simulink model "k1visitmyp"  (Simulink 8.8)
settings: Solver=ode45  StartTime=0.0  StopTime=10.0  RelTol=1e-3  EnableMultiTasking=on
libraries: cdsIPCx x26, cdsCDI64 x6, cdsCDO64 x6, BIO_CD_DECODE_MASTER x6, BIO_CD_ENCODE_MASTER x5, CHK_DIO x5, dac x3, cdsBit2Word x2, cdsAdcx0 x1, cdsAdcx1 x1, TYPEA_MASTER x1, cdsEpicsOut x1
settings Model: SuppressorTable=22 serialization::archive 11 0 3 0 0 0 11 0  Creator=controls  LastModifiedBy=controls
settings DataIOCC: SignalLoggingSaveFormat=Dataset
settings DebuggingCC: UnderspecifiedInitializationDetection=Simplified  MergeDetectMultiDrivingBlocksExec=error  FcnCallInpInsideContextMsg=error  AllowSymbolicDim=off  StateNameClashWarn=none
settings GRTTargetCC: CombineOutputUpdateFcns=on  GRTInterface=off

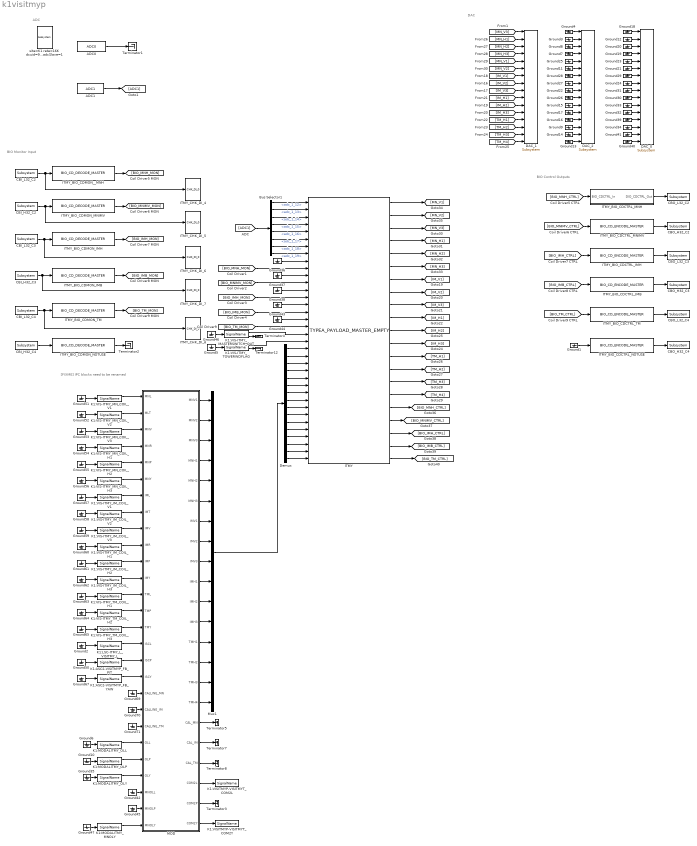
== system k1visitmyp ==
  note: [FIXME] IPC blocks need to be renamed
  note: BIO Monitor Input
  note: BIO Control Outputs
  note: DAC
  note: ADC
  ADC0 : cdsAdcx0/ADC0  Tag=cdsAdc  Description=|
      | type-GSC_16AI64SSA
      | card_num=0
      settings: AttributesFormatString=%<Description>\n%<Tag>
  ADC1 : cdsAdcx1/ADC1  Tag=cdsAdc  Description=|
      | type-GSC_16AI64SSA
      | card_num=1
      settings: AttributesFormatString=%<Description>\n%<Tag>
  Bus Selector1 : BusSelector  OutputSignals=adc_1_12,adc_1_13,adc_1_14,adc_1_15,adc_1_16,adc_1_17,adc_1_18,adc_1_19
  CBI_H32_C2 : cdsCDI64/Subsystem  Tag=cdsCDI64  Description=card_num=5
      settings: AttributesFormatString=%<Tag>\n%<Description>
  CBI_H32_C3 : cdsCDI64/Subsystem  Tag=cdsCDI64  Description=card_num=7
      settings: AttributesFormatString=%<Tag>\n%<Description>
  CBI_H32_C4 : cdsCDI64/Subsystem  Tag=cdsCDI64  Description=card_num=9
      settings: AttributesFormatString=%<Tag>\n%<Description>
  CBI_L32_C2 : cdsCDI64/Subsystem  Tag=cdsCDI64  Description=card_num=4
      settings: AttributesFormatString=%<Tag>\n%<Description>
  CBI_L32_C3 : cdsCDI64/Subsystem  Tag=cdsCDI64  Description=card_num=6
      settings: AttributesFormatString=%<Tag>\n%<Description>
  CBI_L32_C4 : cdsCDI64/Subsystem  Tag=cdsCDI64  Description=card_num=8
      settings: AttributesFormatString=%<Tag>\n%<Description>
  CBO_H32_C2 : cdsCDO64/Subsystem  Tag=cdsCDO64  Description=card_num=5
      settings: AttributesFormatString=%<Tag>\n%<Description>
  CBO_H32_C3 : cdsCDO64/Subsystem  Tag=cdsCDO64  Description=card_num=7
      settings: AttributesFormatString=%<Tag>\n%<Description>
  CBO_H32_C4 : cdsCDO64/Subsystem  Tag=cdsCDO64  Description=card_num=9
      settings: AttributesFormatString=%<Tag>\n%<Description>
  CBO_L32_C2 : cdsCDO64/Subsystem  Tag=cdsCDO64  Description=card_num=4
      settings: AttributesFormatString=%<Tag>\n%<Description>
  CBO_L32_C3 : cdsCDO64/Subsystem  Tag=cdsCDO64  Description=card_num=6
      settings: AttributesFormatString=%<Tag>\n%<Description>
  CBO_L32_C4 : cdsCDO64/Subsystem  Tag=cdsCDO64  Description=card_num=8
      settings: AttributesFormatString=%<Tag>\n%<Description>
  DAC_0 : dac/Subsystem  Description=|
      | type=GSC_16AO16,
      | card_num=0
      settings: AttributesFormatString=%<Description>
  DAC_1 : dac/Subsystem  Description=|
      | type=GSC_16AO16,
      | card_num=1
      settings: AttributesFormatString=%<Description>
  DAC_2 : dac/Subsystem  Description=|
      | type=GSC_16AO16,
      | card_num=2
      settings: AttributesFormatString=%<Description>
  Demux : Demux  Outputs=16
  Ground{1..47,50..65,67,69..71} (67 alike) : Ground
  ITMY : TYPEA_MASTER/TYPEA_PAYLOAD_MASTER_EMPTY
  ITMY_BIO_CDCTRL_IMB : BIO_CD_ENCODE_MASTER/BIO_CD_ENCODE_MASTER
  ITMY_BIO_CDCTRL_IMH : BIO_CD_ENCODE_MASTER/BIO_CD_ENCODE_MASTER
  ITMY_BIO_CDCTRL_MNH : Subsystem
  ITMY_BIO_CDCTRL_MNIMV : BIO_CD_ENCODE_MASTER/BIO_CD_ENCODE_MASTER
  ITMY_BIO_CDCTRL_NOTUSE : BIO_CD_ENCODE_MASTER/BIO_CD_ENCODE_MASTER
  ITMY_BIO_CDCTRL_TM : BIO_CD_ENCODE_MASTER/BIO_CD_ENCODE_MASTER
  ITMY_BIO_CDMON_IMB : BIO_CD_DECODE_MASTER/BIO_CD_DECODE_MASTER
  ITMY_BIO_CDMON_IMH : BIO_CD_DECODE_MASTER/BIO_CD_DECODE_MASTER
  ITMY_BIO_CDMON_MNIMV : BIO_CD_DECODE_MASTER/BIO_CD_DECODE_MASTER
  ITMY_BIO_CDMON_NOTUSE : BIO_CD_DECODE_MASTER/BIO_CD_DECODE_MASTER
  ITMY_BIO_CDMON_TM : BIO_CD_DECODE_MASTER/BIO_CD_DECODE_MASTER
  ITMY_BIO_CDMON__MNH : BIO_CD_DECODE_MASTER/BIO_CD_DECODE_MASTER
  ITMY_CHK_DI_{4..8} (5 alike) : CHK_DIO/CHK_DI_0
  K1:ASC2-VISITMYP_FB_PIT : cdsIPCx/SignalName  Tag=cdsIPCx_RFM  Description=card=1
      settings: AttributesFormatString=%<Description>\n%<Tag>
  K1:ASC2-VISITMYP_FB_YAW : cdsIPCx/SignalName  Tag=cdsIPCx_RFM  Description=card=1
      settings: AttributesFormatString=%<Description>\n%<Tag>
  K1:LSC-ITMY_L_VISITMY_L : cdsIPCx/SignalName  Tag=cdsIPCx_RFM  Description=card=1
      settings: AttributesFormatString=%<Description>\n%<Tag>
  K1:MODALITMY_MNOLY : cdsIPCx/SignalName  Tag=cdsIPCx_SHMEM  Description=Inter-Process Communication via Shared memory.
      settings: AttributesFormatString=%<Tag>
  K1:MODALITMY_OLL : cdsIPCx/SignalName  Tag=cdsIPCx_SHMEM  Description=Inter-Process Communication via Shared memory.
      settings: AttributesFormatString=%<Tag>
  K1:MODALITMY_OLP : cdsIPCx/SignalName  Tag=cdsIPCx_SHMEM  Description=Inter-Process Communication via Shared memory.
      settings: AttributesFormatString=%<Tag>
  K1:MODALITMY_OLY : cdsIPCx/SignalName  Tag=cdsIPCx_SHMEM  Description=Inter-Process Communication via Shared memory.
      settings: AttributesFormatString=%<Tag>
  K1:VIS-ITMY_IM_COIL_H1 : cdsIPCx/SignalName  Tag=cdsIPCx_SHMEM  Description=Inter-Process Communication via Shared memory.
      settings: AttributesFormatString=%<Tag>
  K1:VIS-ITMY_IM_COIL_H2 : cdsIPCx/SignalName  Tag=cdsIPCx_SHMEM  Description=Inter-Process Communication via Shared memory.
      settings: AttributesFormatString=%<Tag>
  K1:VIS-ITMY_IM_COIL_H3 : cdsIPCx/SignalName  Tag=cdsIPCx_SHMEM  Description=Inter-Process Communication via Shared memory.
      settings: AttributesFormatString=%<Tag>
  K1:VIS-ITMY_IM_COIL_V1 : cdsIPCx/SignalName  Tag=cdsIPCx_SHMEM  Description=Inter-Process Communication via Shared memory.
      settings: AttributesFormatString=%<Tag>
  K1:VIS-ITMY_IM_COIL_V2 : cdsIPCx/SignalName  Tag=cdsIPCx_SHMEM  Description=Inter-Process Communication via Shared memory.
      settings: AttributesFormatString=%<Tag>
  K1:VIS-ITMY_IM_COIL_V3 : cdsIPCx/SignalName  Tag=cdsIPCx_SHMEM  Description=Inter-Process Communication via Shared memory.
      settings: AttributesFormatString=%<Tag>
  K1:VIS-ITMY_MASTERSWITCH_OUT : cdsIPCx/SignalName  Tag=cdsIPCx_SHMEM  Description=Inter-Process Communication via Shared memory.
      settings: AttributesFormatString=%<Tag>
  K1:VIS-ITMY_MN_COIL_H1 : cdsIPCx/SignalName  Tag=cdsIPCx_SHMEM  Description=Inter-Process Communication via Shared memory.
      settings: AttributesFormatString=%<Tag>
  K1:VIS-ITMY_MN_COIL_H2 : cdsIPCx/SignalName  Tag=cdsIPCx_SHMEM  Description=Inter-Process Communication via Shared memory.
      settings: AttributesFormatString=%<Tag>
  K1:VIS-ITMY_MN_COIL_H3 : cdsIPCx/SignalName  Tag=cdsIPCx_SHMEM  Description=Inter-Process Communication via Shared memory.
      settings: AttributesFormatString=%<Tag>
  K1:VIS-ITMY_MN_COIL_V1 : cdsIPCx/SignalName  Tag=cdsIPCx_SHMEM  Description=Inter-Process Communication via Shared memory.
      settings: AttributesFormatString=%<Tag>
  K1:VIS-ITMY_MN_COIL_V2 : cdsIPCx/SignalName  Tag=cdsIPCx_SHMEM  Description=Inter-Process Communication via Shared memory.
      settings: AttributesFormatString=%<Tag>
  K1:VIS-ITMY_MN_COIL_V3 : cdsIPCx/SignalName  Tag=cdsIPCx_SHMEM  Description=Inter-Process Communication via Shared memory.
      settings: AttributesFormatString=%<Tag>
  K1:VIS-ITMY_TM_COIL_H1 : cdsIPCx/SignalName  Tag=cdsIPCx_SHMEM  Description=Inter-Process Communication via Shared memory.
      settings: AttributesFormatString=%<Tag>
  K1:VIS-ITMY_TM_COIL_H2 : cdsIPCx/SignalName  Tag=cdsIPCx_SHMEM  Description=Inter-Process Communication via Shared memory.
      settings: AttributesFormatString=%<Tag>
  K1:VIS-ITMY_TM_COIL_H3 : cdsIPCx/SignalName  Tag=cdsIPCx_SHMEM  Description=Inter-Process Communication via Shared memory.
      settings: AttributesFormatString=%<Tag>
  K1:VIS-ITMY_TOWERWDFLAG : cdsIPCx/SignalName  Tag=cdsIPCx_SHMEM  Description=Inter-Process Communication via Shared memory.
      settings: AttributesFormatString=%<Tag>
  K1:VISITMYP-VISITMYT_COM2L : cdsIPCx/SignalName  Tag=cdsIPCx_SHMEM  Description=Inter-Process Communication via Shared memory.
      settings: AttributesFormatString=%<Tag>
  K1:VISITMYP-VISITMYT_COM2Y : cdsIPCx/SignalName  Tag=cdsIPCx_SHMEM  Description=Inter-Process Communication via Shared memory.
      settings: AttributesFormatString=%<Tag>
  MOD : Subsystem  Tag=top_names
  Mux1 : Mux  Inputs=16
  Terminator{1..5,7..8,12} (8 alike) : Terminator
  site=K1 rate=16K dcuid=98 host=k1iy1 specific_cpu=3 adcSlave=1 : cdsParameters/Subsystem  Tag=cdsParameters  Description=|
      | Purpose:                                                                                                                                                                                                                                
      | Provide system parameters to the FE code generator to properly configure the generated EPICS names, rep rate of the FE controller, and the Data Acquisition node ID for proper storage of data from this FE controller.                 
      |                                                                                                                                                                                                                                         
      | Useage:                                                                                                                                                                                                                                 
      | The part NAME field is used to identify the FE parameters. It must be of the form:                                                                                                                                                      
      | site=                                                                                                                                                                                                                                   
      | rate=                                                                                                                                                                                                                                   
      | dcuid=                                                                                                                                                                                                                                  
      |                                                                                                                                                                                                                                         
      | Where:                                                                                                                                                                                                                                  
      | site= argument may be H1, H2, L1, M1, G1, either as a single argument or multiple, for example site=H1,H2. These are the only names allowed. These will become the first two characters of all EPICS and signal names (for example G1:).
      |                                                                                                                                                                                                                                         
      | rate= may be 2K, 16K, 32K, or 64K                                                                                                                                                                                                       
      |                                                                                                                                                                                                                                         
      | dcuid= is site specific ie it must be unique at each site.
      settings: AttributesFormatString=%<Tag>
  wires:
  ADC1/1 -> [ADC1]
  [MN_V3] -> DAC_1/1
  [MN_H1] -> DAC_1/2
  [MN_H2] -> DAC_1/3
  [MN_H3] -> DAC_1/4
  [MN_V1] -> DAC_1/5
  [MN_V2] -> DAC_1/6
  [IM_V1] -> DAC_1/7
  [IM_V2] -> DAC_1/8
  [IM_V3] -> DAC_1/9
  [IM_H1] -> DAC_1/10
  [TM_H1] -> DAC_1/13
  [TM_H4] -> DAC_1/16
  [TM_H3] -> DAC_1/15
  [TM_H2] -> DAC_1/14
  [IM_H2] -> DAC_1/11
  [IM_H3] -> DAC_1/12
  [BIO_MNH_CTRL] -> ITMY_BIO_CDCTRL_MNH/1(BIO_CDCTRL_In)
  ITMY_BIO_CDCTRL_MNH/1(DIO_CDCTRL_Out) -> CBO_L32_C2/1
  [BIO_MNIMV_CTRL] -> ITMY_BIO_CDCTRL_MNIMV/1
  ITMY_BIO_CDCTRL_MNIMV/1 -> CBO_H32_C2/1
  [BIO_IMH_CTRL] -> ITMY_BIO_CDCTRL_IMH/1
  ITMY_BIO_CDCTRL_IMH/1 -> CBO_L32_C3/1
  [BIO_IMB_CTRL] -> ITMY_BIO_CDCTRL_IMB/1
  ITMY_BIO_CDCTRL_IMB/1 -> CBO_H32_C3/1
  [BIO_TM_CTRL] -> ITMY_BIO_CDCTRL_TM/1
  ITMY_BIO_CDCTRL_TM/1 -> CBO_L32_C4/1
  Ground1/1 -> ITMY_BIO_CDCTRL_NOTUSE/1
  ITMY_BIO_CDCTRL_NOTUSE/1 -> CBO_H32_C4/1
  CBI_L32_C2/1 -> ITMY_CHK_DI_4/1, ITMY_BIO_CDMON__MNH/1
  ITMY_BIO_CDMON__MNH/1 -> [BIO_MNH_MON]
  CBI_H32_C2/1 -> ITMY_CHK_DI_5/1, ITMY_BIO_CDMON_MNIMV/1
  ITMY_BIO_CDMON_MNIMV/1 -> [BIO_MNIMV_MON]
  CBI_L32_C3/1 -> ITMY_CHK_DI_6/1, ITMY_BIO_CDMON_IMH/1
  ITMY_BIO_CDMON_IMH/1 -> [BIO_IMH_MON]
  ITMY_BIO_CDMON_IMB/1 -> [BIO_IMB_MON]
  CBI_L32_C4/1 -> ITMY_CHK_DI_8/1, ITMY_BIO_CDMON_TM/1
  ITMY_BIO_CDMON_TM/1 -> [BIO_TM_MON]
  CBI_H32_C4/1 -> ITMY_BIO_CDMON_NOTUSE/1
  ITMY_BIO_CDMON_NOTUSE/1 -> Terminator2/1
  Ground4/1 -> DAC_2/1
  Ground3/1 -> DAC_2/2
  Ground8/1 -> DAC_2/3
  Ground7/1 -> DAC_2/4
  Ground25/1 -> DAC_2/5
  Ground11/1 -> DAC_2/6
  Ground28/1 -> DAC_2/7
  Ground27/1 -> DAC_2/8
  Ground22/1 -> DAC_2/9
  Ground26/1 -> DAC_2/10
  Ground15/1 -> DAC_2/11
  Ground17/1 -> DAC_2/12
  Ground16/1 -> DAC_2/13
  Ground9/1 -> DAC_2/14
  Ground14/1 -> DAC_2/15
  Ground13/1 -> DAC_2/16
  CBI_H32_C3/1 -> ITMY_CHK_DI_7/1, ITMY_BIO_CDMON_IMB/1
  [ADC1] -> Bus Selector1/1
  K1:VIS-ITMY_TOWERWDFLAG/2 -> Terminator12/1
  Ground5/1 -> K1:VIS-ITMY_TOWERWDFLAG/1
  ADC0/1 -> Terminator1/1
  Ground18/1 -> DAC_0/1
  Ground12/1 -> DAC_0/2
  Ground19/1 -> DAC_0/4
  Ground20/1 -> DAC_0/3
  Ground29/1 -> DAC_0/7
  Ground23/1 -> DAC_0/5
  Ground21/1 -> DAC_0/6
  Ground24/1 -> DAC_0/8
  Ground31/1 -> DAC_0/9
  Ground30/1 -> DAC_0/10
  Ground33/1 -> DAC_0/11
  Ground32/1 -> DAC_0/12
  Ground39/1 -> DAC_0/13
  Ground34/1 -> DAC_0/14
  Ground41/1 -> DAC_0/15
  Ground40/1 -> DAC_0/16
  Ground2/1 -> K1:LSC-ITMY_L_VISITMY_L/1
  Ground46/1 -> K1:VIS-ITMY_MASTERSWITCH_OUT/1
  K1:VIS-ITMY_MASTERSWITCH_OUT/2 -> Terminator4/1
  Ground36/1 -> ITMY/9
  [BIO_MNH_MON] -> ITMY/10
  Ground37/1 -> ITMY/11
  [BIO_MNIMV_MON] -> ITMY/12
  Ground38/1 -> ITMY/13
  [BIO_IMH_MON] -> ITMY/14
  Ground43/1 -> ITMY/15
  [BIO_IMB_MON] -> ITMY/16
  Ground44/1 -> ITMY/17
  [BIO_TM_MON] -> ITMY/18
  ITMY/2 -> [MN_V2]
  ITMY/1 -> [MN_V1]
  ITMY/3 -> [MN_V3]
  ITMY/4 -> [MN_H1]
  ITMY/5 -> [MN_H2]
  ITMY/6 -> [MN_H3]
  ITMY/7 -> [IM_V1]
  ITMY/8 -> [IM_V2]
  ITMY/9 -> [IM_V3]
  ITMY/10 -> [IM_H1]
  ITMY/11 -> [IM_H2]
  ITMY/12 -> [IM_H3]
  ITMY/13 -> [TM_H1]
  ITMY/14 -> [TM_H2]
  ITMY/15 -> [TM_H3]
  ITMY/19 -> [BIO_IMH_CTRL]
  ITMY/18 -> [BIO_MNIMV_CTRL]
  ITMY/17 -> [BIO_MNH_CTRL]
  ITMY/16 -> [TM_H4]
  Mux1/1 -> Demux/1
  ITMY/20 -> [BIO_IMB_CTRL]
  ITMY/21 -> [BIO_TM_CTRL]
  Ground51/1 -> K1:VIS-ITMY_MN_COIL_V1/1
  Ground52/1 -> K1:VIS-ITMY_MN_COIL_V2/1
  Ground53/1 -> K1:VIS-ITMY_MN_COIL_V3/1
  Ground54/1 -> K1:VIS-ITMY_MN_COIL_H1/1
  Ground55/1 -> K1:VIS-ITMY_MN_COIL_H2/1
  Ground56/1 -> K1:VIS-ITMY_MN_COIL_H3/1
  Ground57/1 -> K1:VIS-ITMY_IM_COIL_V1/1
  Ground58/1 -> K1:VIS-ITMY_IM_COIL_V2/1
  Ground59/1 -> K1:VIS-ITMY_IM_COIL_V3/1
  Ground60/1 -> K1:VIS-ITMY_IM_COIL_H1/1
  Ground61/1 -> K1:VIS-ITMY_IM_COIL_H2/1
  Ground62/1 -> K1:VIS-ITMY_IM_COIL_H3/1
  Ground63/1 -> K1:VIS-ITMY_TM_COIL_H1/1
  Ground64/1 -> K1:VIS-ITMY_TM_COIL_H2/1
  Ground65/1 -> K1:VIS-ITMY_TM_COIL_H3/1
  K1:VIS-ITMY_MN_COIL_V1/1 -> MOD/1(MNL)
  K1:VIS-ITMY_MN_COIL_V2/1 -> MOD/2(MLT)
  K1:VIS-ITMY_MN_COIL_V3/1 -> MOD/3(MNV)
  K1:VIS-ITMY_MN_COIL_H1/1 -> MOD/4(MNR)
  K1:VIS-ITMY_MN_COIL_H2/1 -> MOD/5(MNP)
  K1:VIS-ITMY_MN_COIL_H3/1 -> MOD/6(MNY)
  K1:VIS-ITMY_IM_COIL_V1/1 -> MOD/7(IML)
  K1:VIS-ITMY_IM_COIL_V2/1 -> MOD/8(IMT)
  K1:VIS-ITMY_IM_COIL_V3/1 -> MOD/9(IMV)
  K1:VIS-ITMY_IM_COIL_H1/1 -> MOD/10(IMR)
  K1:VIS-ITMY_IM_COIL_H2/1 -> MOD/11(IMP)
  K1:VIS-ITMY_IM_COIL_H3/1 -> MOD/12(IMY)
  K1:VIS-ITMY_TM_COIL_H1/1 -> MOD/13(TML)
  K1:VIS-ITMY_TM_COIL_H2/1 -> MOD/14(TMP)
  K1:VIS-ITMY_TM_COIL_H3/1 -> MOD/15(TMY)
  MOD/1(MNV1) -> Mux1/1
  MOD/2(MNV2) -> Mux1/2
  MOD/3(MNV3) -> Mux1/3
  MOD/4(MNH1) -> Mux1/4
  MOD/5(MNH2) -> Mux1/5
  MOD/6(MNH3) -> Mux1/6
  MOD/7(IMV1) -> Mux1/7
  MOD/8(IMV2) -> Mux1/8
  MOD/9(IMV3) -> Mux1/9
  MOD/10(IMH1) -> Mux1/10
  MOD/11(IMH2) -> Mux1/11
  MOD/12(IMH3) -> Mux1/12
  MOD/13(TMH1) -> Mux1/13
  MOD/14(TMH2) -> Mux1/14
  MOD/15(TMH3) -> Mux1/15
  MOD/16(TMH4) -> Mux1/16
  K1:LSC-ITMY_L_VISITMY_L/1 -> MOD/16(ISCL)
  Ground69/1 -> MOD/19(CALLINE_MN)
  Ground70/1 -> MOD/20(CALLINE_IM)
  Ground71/1 -> MOD/21(CALLINE_TM)
  MOD/19(CAL_TM) -> Terminator8/1
  MOD/18(CAL_IM) -> Terminator7/1
  MOD/17(CAL_MN) -> Terminator5/1
  Demux/2 -> ITMY/22
  Demux/3 -> ITMY/23
  Demux/4 -> ITMY/24
  Demux/5 -> ITMY/25
  Demux/6 -> ITMY/26
  Demux/7 -> ITMY/27
  Demux/8 -> ITMY/28
  Demux/9 -> ITMY/29
  Demux/10 -> ITMY/30
  Demux/11 -> ITMY/31
  Demux/12 -> ITMY/32
  Demux/13 -> ITMY/33
  Demux/14 -> ITMY/34
  Demux/15 -> ITMY/35
  Demux/16 -> ITMY/36
  Demux/1 -> ITMY/21
  K1:ASC2-VISITMYP_FB_PIT/1 -> MOD/17(ISCP)
  K1:ASC2-VISITMYP_FB_YAW/1 -> MOD/18(ISCY)
  Ground50/1 -> K1:ASC2-VISITMYP_FB_PIT/1
  Ground67/1 -> K1:ASC2-VISITMYP_FB_YAW/1
  Bus Selector1/1 -> ITMY/1  "<adc_1_12>"
  Bus Selector1/2 -> ITMY/2  "<adc_1_13>"
  Bus Selector1/3 -> ITMY/3  "<adc_1_14>"
  Bus Selector1/4 -> ITMY/4  "<adc_1_15>"
  Bus Selector1/5 -> ITMY/5  "<adc_1_16>"
  Bus Selector1/6 -> ITMY/6  "<adc_1_17>"
  Bus Selector1/7 -> ITMY/7  "<adc_1_18>"
  Bus Selector1/8 -> ITMY/8  "<adc_1_19>"
  K1:VIS-ITMY_TOWERWDFLAG/1 -> ITMY/20
  K1:VIS-ITMY_MASTERSWITCH_OUT/1 -> ITMY/19
  MOD/20(COM2L) -> K1:VISITMYP-VISITMYT_COM2L/1
  MOD/22(COM2Y) -> K1:VISITMYP-VISITMYT_COM2Y/1
  MOD/21(COM2P) -> Terminator3/1
  K1:MODALITMY_OLL/1 -> MOD/22(OLL)
  K1:MODALITMY_OLP/1 -> MOD/23(OLP)
  K1:MODALITMY_OLY/1 -> MOD/24(OLY)
  Ground35/1 -> K1:MODALITMY_OLY/1
  Ground6/1 -> K1:MODALITMY_OLL/1
  Ground10/1 -> K1:MODALITMY_OLP/1
  Ground42/1 -> MOD/25(MNOLL)
  Ground45/1 -> MOD/26(MNOLP)
  K1:MODALITMY_MNOLY/1 -> MOD/27(MNOLY)
  Ground47/1 -> K1:MODALITMY_MNOLY/1

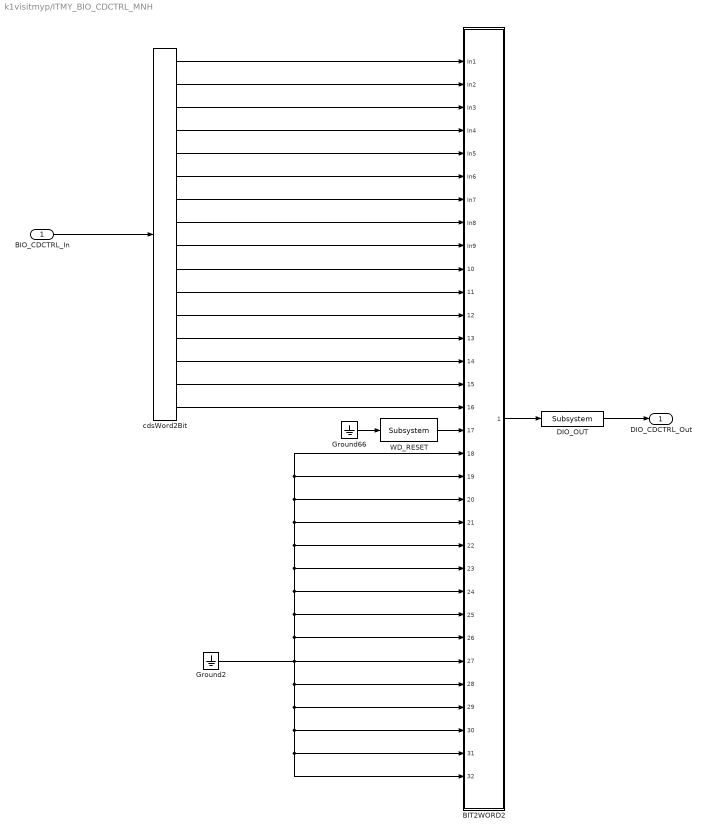
== system k1visitmyp/ITMY_BIO_CDCTRL_MNH ==
  BIO_CDCTRL_In : Inport
  BIT2WORD2 : Subsystem
  DIO_OUT : cdsEpicsOut/Subsystem  Tag=cdsEpicsOutput  Description=|
      | Purpose:                                          
      | Output a FE signal to an EPICS channel.           
      |                                                   
      | Operation:                                        
      | Takes input value and passes it to EPICS record.  
      |                                                   
      | Usage:                                            
      | Name the part with the desired EPICS rrecord name.
      settings: AttributesFormatString=%<Tag>
  Ground2 : Ground
  Ground66 : Ground
  WD_RESET : cdsEpicsBinIn/Subsystem  Tag=cdsEpicsBinIn  Description=|
      | Purpose:                                                                            
      | Create an EPICS binary (0 or 1) input channel to the FE realtime controls.          
      |                                                                                     
      | Operation:                                                                          
      | Outputs value from an EPICS ai record. Value is binary input (bi Epics record type).
      |                                                                                     
      | Usage:                                                                              
      | Name the part with the desired EPICS channel name.
      settings: AttributesFormatString=%<Tag>
  cdsWord2Bit : cdsWord2Bit/cdsWord2Bit  Tag=cdsWord2Bit  Description=Generate 16 0/1 outputs from single 16-bit integer input
      settings: AttributesFormatString=cdsWord2Bit
  DIO_CDCTRL_Out : Outport
  wires:
  BIT2WORD2/1(Out1) -> DIO_OUT/1
  DIO_OUT/1 -> DIO_CDCTRL_Out/1
  BIO_CDCTRL_In/1 -> cdsWord2Bit/1
  cdsWord2Bit/1 -> BIT2WORD2/1(In1)
  cdsWord2Bit/2 -> BIT2WORD2/2(In2)
  cdsWord2Bit/3 -> BIT2WORD2/3(In3)
  cdsWord2Bit/4 -> BIT2WORD2/4(In4)
  cdsWord2Bit/5 -> BIT2WORD2/5(In5)
  cdsWord2Bit/6 -> BIT2WORD2/6(In6)
  cdsWord2Bit/7 -> BIT2WORD2/7(In7)
  cdsWord2Bit/8 -> BIT2WORD2/8(In8)
  cdsWord2Bit/9 -> BIT2WORD2/9(In9)
  cdsWord2Bit/10 -> BIT2WORD2/10(In10)
  cdsWord2Bit/11 -> BIT2WORD2/11(In11)
  cdsWord2Bit/12 -> BIT2WORD2/12(In12)
  cdsWord2Bit/13 -> BIT2WORD2/13(In13)
  cdsWord2Bit/14 -> BIT2WORD2/14(In14)
  cdsWord2Bit/15 -> BIT2WORD2/15(In15)
  cdsWord2Bit/16 -> BIT2WORD2/16(In16)
  WD_RESET/1 -> BIT2WORD2/17(In17)
  Ground66/1 -> WD_RESET/1
  Ground2/1 -> BIT2WORD2/27(In27), BIT2WORD2/28(In28), BIT2WORD2/29(In29), BIT2WORD2/30(In30), BIT2WORD2/31(In31), BIT2WORD2/32(In32), BIT2WORD2/26(In26), BIT2WORD2/25(In25), BIT2WORD2/24(In24), BIT2WORD2/23(In23), BIT2WORD2/22(In22), BIT2WORD2/21(In21), BIT2WORD2/20(In20), BIT2WORD2/18(In18), BIT2WORD2/19(In19)

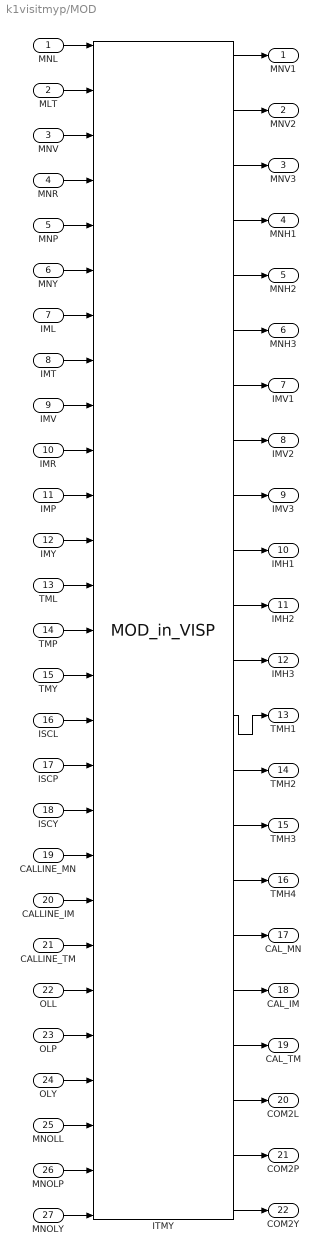
== system k1visitmyp/MOD ==
  MNL : Inport
  MLT : Inport  Port=2
  MNV : Inport  Port=3
  MNR : Inport  Port=4
  MNP : Inport  Port=5
  MNY : Inport  Port=6
  IML : Inport  Port=7
  IMT : Inport  Port=8
  IMV : Inport  Port=9
  IMR : Inport  Port=10
  IMP : Inport  Port=11
  IMY : Inport  Port=12
  TML : Inport  Port=13
  TMP : Inport  Port=14
  TMY : Inport  Port=15
  ISCL : Inport  Port=16
  ISCP : Inport  Port=17
  ISCY : Inport  Port=18
  CALLINE_MN : Inport  Port=19
  CALLINE_IM : Inport  Port=20
  CALLINE_TM : Inport  Port=21
  OLL : Inport  Port=22
  OLP : Inport  Port=23
  OLY : Inport  Port=24
  MNOLL : Inport  Port=25
  MNOLP : Inport  Port=26
  MNOLY : Inport  Port=27
  ITMY : VIS_LIB/MODAL/MOD_in_VISP  Tag=top_names
  MNV1 : Outport
  MNV2 : Outport  Port=2
  MNV3 : Outport  Port=3
  MNH1 : Outport  Port=4
  MNH2 : Outport  Port=5
  MNH3 : Outport  Port=6
  IMV1 : Outport  Port=7
  IMV2 : Outport  Port=8
  IMV3 : Outport  Port=9
  IMH1 : Outport  Port=10
  IMH2 : Outport  Port=11
  IMH3 : Outport  Port=12
  TMH1 : Outport  Port=13
  TMH2 : Outport  Port=14
  TMH3 : Outport  Port=15
  TMH4 : Outport  Port=16
  CAL_MN : Outport  Port=17
  CAL_IM : Outport  Port=18
  CAL_TM : Outport  Port=19
  COM2L : Outport  Port=20
  COM2P : Outport  Port=21
  COM2Y : Outport  Port=22
  wires:
  MNL/1 -> ITMY/1
  TMY/1 -> ITMY/15
  MLT/1 -> ITMY/2
  MNV/1 -> ITMY/3
  MNR/1 -> ITMY/4
  MNP/1 -> ITMY/5
  MNY/1 -> ITMY/6
  IML/1 -> ITMY/7
  IMT/1 -> ITMY/8
  IMV/1 -> ITMY/9
  IMR/1 -> ITMY/10
  IMP/1 -> ITMY/11
  IMY/1 -> ITMY/12
  TML/1 -> ITMY/13
  TMP/1 -> ITMY/14
  ITMY/1 -> MNV1/1
  ITMY/16 -> TMH4/1
  ITMY/2 -> MNV2/1
  ITMY/3 -> MNV3/1
  ITMY/4 -> MNH1/1
  ITMY/5 -> MNH2/1
  ITMY/6 -> MNH3/1
  ITMY/7 -> IMV1/1
  ITMY/8 -> IMV2/1
  ITMY/9 -> IMV3/1
  ITMY/10 -> IMH1/1
  ITMY/11 -> IMH2/1
  ITMY/12 -> IMH3/1
  ITMY/13 -> TMH1/1
  ITMY/14 -> TMH2/1
  ITMY/15 -> TMH3/1
  ISCL/1 -> ITMY/16
  CALLINE_TM/1 -> ITMY/21
  CALLINE_IM/1 -> ITMY/20
  CALLINE_MN/1 -> ITMY/19
  ISCP/1 -> ITMY/17
  ISCY/1 -> ITMY/18
  ITMY/17 -> CAL_MN/1
  ITMY/18 -> CAL_IM/1
  ITMY/19 -> CAL_TM/1
  ITMY/22 -> COM2Y/1
  ITMY/21 -> COM2P/1
  ITMY/20 -> COM2L/1
  OLY/1 -> ITMY/24
  OLP/1 -> ITMY/23
  OLL/1 -> ITMY/22
  MNOLY/1 -> ITMY/27
  MNOLP/1 -> ITMY/26
  MNOLL/1 -> ITMY/25

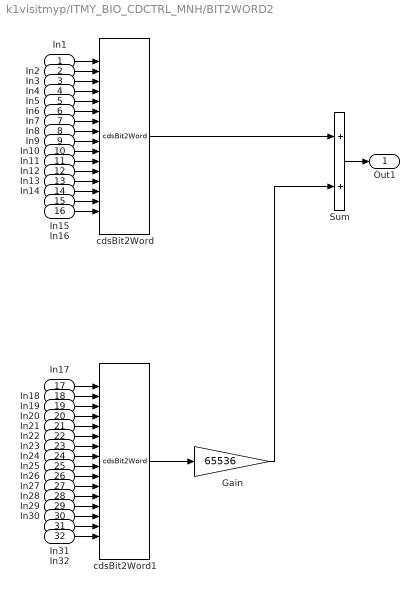
== system k1visitmyp/ITMY_BIO_CDCTRL_MNH/BIT2WORD2 ==
  In1 : Inport
  In2 : Inport  Port=2
  In3 : Inport  Port=3
  In4 : Inport  Port=4
  In5 : Inport  Port=5
  In6 : Inport  Port=6
  In7 : Inport  Port=7
  In8 : Inport  Port=8
  In9 : Inport  Port=9
  In10 : Inport  Port=10
  In11 : Inport  Port=11
  In12 : Inport  Port=12
  In13 : Inport  Port=13
  In14 : Inport  Port=14
  In15 : Inport  Port=15
  In16 : Inport  Port=16
  In17 : Inport  Port=17
  In18 : Inport  Port=18
  In19 : Inport  Port=19
  In20 : Inport  Port=20
  In21 : Inport  Port=21
  In22 : Inport  Port=22
  In23 : Inport  Port=23
  In24 : Inport  Port=24
  In25 : Inport  Port=25
  In26 : Inport  Port=26
  In27 : Inport  Port=27
  In28 : Inport  Port=28
  In29 : Inport  Port=29
  In30 : Inport  Port=30
  In31 : Inport  Port=31
  In32 : Inport  Port=32
  Gain : Gain  Gain=65536
  Sum : Sum
  cdsBit2Word : cdsBit2Word/cdsBit2Word  Tag=cdsBit2Word  Description=Forms single 16 bit integer from 16 0/1 inputs.
      settings: AttributesFormatString=%<Tag>
  cdsBit2Word1 : cdsBit2Word/cdsBit2Word  Tag=cdsBit2Word  Description=Forms single 16 bit integer from 16 0/1 inputs.
      settings: AttributesFormatString=%<Tag>
  Out1 : Outport
  wires:
  In32/1 -> cdsBit2Word1/16
  In31/1 -> cdsBit2Word1/15
  In30/1 -> cdsBit2Word1/14
  In29/1 -> cdsBit2Word1/13
  In28/1 -> cdsBit2Word1/12
  In27/1 -> cdsBit2Word1/11
  In26/1 -> cdsBit2Word1/10
  In25/1 -> cdsBit2Word1/9
  In24/1 -> cdsBit2Word1/8
  In23/1 -> cdsBit2Word1/7
  In22/1 -> cdsBit2Word1/6
  In21/1 -> cdsBit2Word1/5
  In20/1 -> cdsBit2Word1/4
  In19/1 -> cdsBit2Word1/3
  In18/1 -> cdsBit2Word1/2
  In17/1 -> cdsBit2Word1/1
  In16/1 -> cdsBit2Word/16
  In15/1 -> cdsBit2Word/15
  In14/1 -> cdsBit2Word/14
  In13/1 -> cdsBit2Word/13
  In12/1 -> cdsBit2Word/12
  In11/1 -> cdsBit2Word/11
  Sum/1 -> Out1/1
  In10/1 -> cdsBit2Word/10
  In9/1 -> cdsBit2Word/9
  In8/1 -> cdsBit2Word/8
  In7/1 -> cdsBit2Word/7
  In6/1 -> cdsBit2Word/6
  In5/1 -> cdsBit2Word/5
  In4/1 -> cdsBit2Word/4
  In3/1 -> cdsBit2Word/3
  In2/1 -> cdsBit2Word/2
  In1/1 -> cdsBit2Word/1
  cdsBit2Word/1 -> Sum/1
  cdsBit2Word1/1 -> Gain/1
  Gain/1 -> Sum/2
